simulink model "myproject_task"  (Simulink 3.00)
libraries: mathlib x8

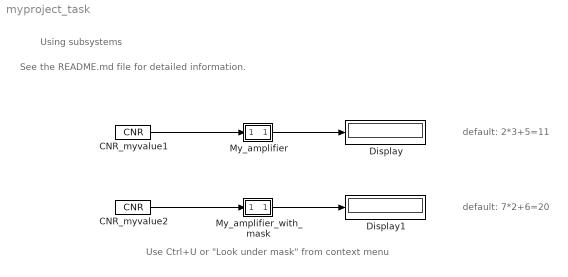
== system myproject_task ==
  note: See the README.md file for detailed information.
  note: Using subsystems
  note: default: 7*2+6=20
  note: default: 2*3+5=11
  note: Use Ctrl+U or
      | "Look under mask"
      | from context menu
  CNR_myvalue1 : mathlib/CNR  ycn=2
  CNR_myvalue2 : mathlib/CNR  ycn=7
  Display : Display
      settings: Format=short
  Display1 : Display
      settings: Format=short
  My_amplifier : Subsystem
      mask Type: REX sequence
  My_amplifier_with_mask : Subsystem  mask(REX sequence){user_gain=2, user_offset=6}
      mask prompts: user_gain "Amplifier gain"; user_offset "Amplifier offset"
  wires:
  CNR_myvalue1/1 -> My_amplifier/1(u)
  CNR_myvalue2/1 -> My_amplifier_with_mask/1(u)
  My_amplifier/1(y) -> Display/1
  My_amplifier_with_mask/1(y) -> Display1/1

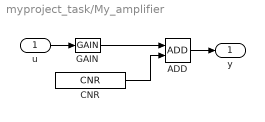
== system myproject_task/My_amplifier ==
  u : Inport  Port=1
  ADD : mathlib/ADD
  CNR : mathlib/CNR  ycn=5
  GAIN : mathlib/GAIN  k=3
  y : Outport  Port=1
  wires:
  ADD/1 -> y/1
  CNR/1 -> ADD/2
  GAIN/1 -> ADD/1
  u/1 -> GAIN/1

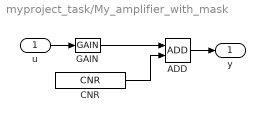
== system myproject_task/My_amplifier_with_mask ==
  u : Inport  Port=1
  ADD : mathlib/ADD
  CNR : mathlib/CNR  ycn=user_offset
  GAIN : mathlib/GAIN  k=user_gain
  y : Outport  Port=1
  wires:
  ADD/1 -> y/1
  CNR/1 -> ADD/2
  GAIN/1 -> ADD/1
  u/1 -> GAIN/1
